simulink model "AOM_new"  (R2023a)
settings: Solver=ode4  StartTime=0.0  StopTime=5  FixedStep=0.001  RelTol=1e-3
values from neighbouring files (symbols this model uses):
  dot_X0 = initial_condition(4:5)    [actor_critic.m]
  trajectory = zeros(4, length(all_new))    [actor_critic.m]
  X0 = initial_condition(1:2)    [actor_critic.m]
libraries: rllib x1
settings Model: Creator=Ali  LastModifiedBy=Ali

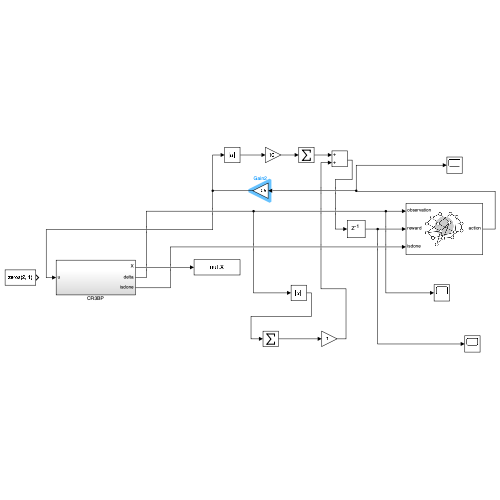
[thumbnail: Simulink's stored preview of the top-level diagram]
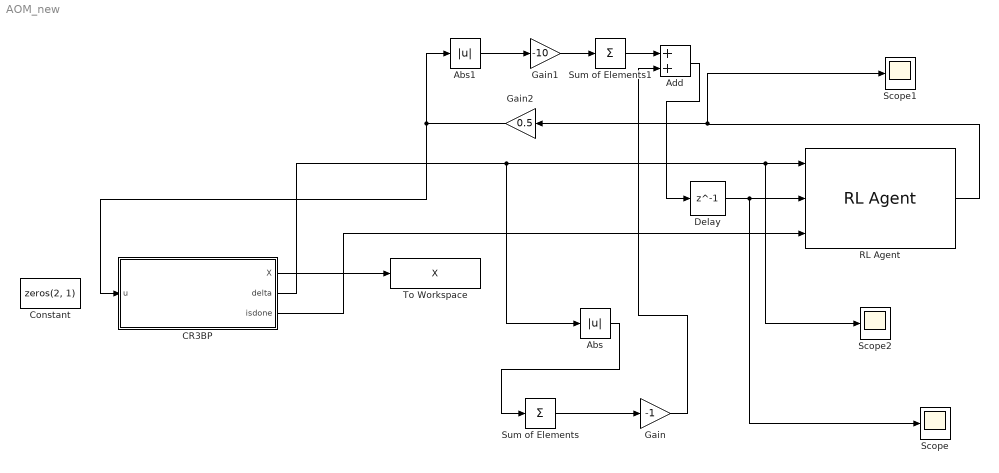
== system AOM_new ==
  Abs : Abs  SaturateOnIntegerOverflow=off
  Abs1 : Abs  SaturateOnIntegerOverflow=off
  Add : Sum
  CR3BP : Subsystem
  Constant : Constant  Value=zeros(2, 1)
  Delay : Delay  DelayLength=1
  Gain : Gain  Gain=-1
  Gain1 : Gain  Gain=-10
  Gain2 : Gain  Gain=0.5
  RL Agent : rllib/RL Agent  Agent=agent2_Trained_3  ExternalActionAsInput=off  ProvideLastAction=off  ProvideCumRwd=off  TreatAsDirectFeedthrough=on  UseStrictObservationDataTypes=off
  Scope : Scope
  Scope1 : Scope
  Scope2 : Scope
  Sum of Elements : Sum  Inputs=+
  Sum of Elements1 : Sum  Inputs=+
  To Workspace : ToWorkspace  VariableName=X  SaveFormat=Timeseries  SampleTime=-1
  wires:
  CR3BP/1(X) -> To Workspace/1
  CR3BP/3(isdone) -> RL Agent/3
  RL Agent/1 -> Gain2/1, Scope1/1
  CR3BP/2(delta) -> Abs/1, Scope2/1, RL Agent/1
  Abs/1 -> Sum of Elements/1
  Sum of Elements/1 -> Gain/1
  Gain/1 -> Add/2
  Delay/1 -> Scope/1, RL Agent/2
  Abs1/1 -> Gain1/1
  Add/1 -> Delay/1
  Sum of Elements1/1 -> Add/1
  Gain1/1 -> Sum of Elements1/1
  Gain2/1 -> CR3BP/1(u), Abs1/1

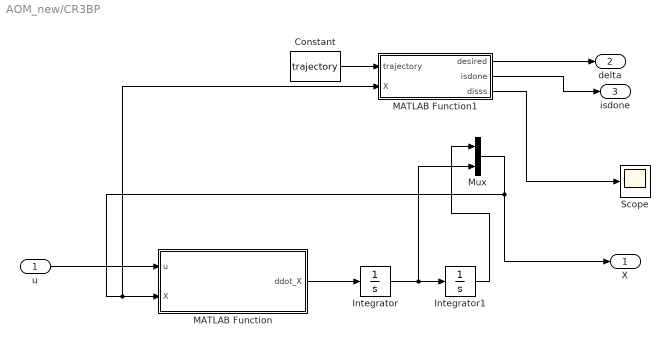
== system AOM_new/CR3BP ==
  u : Inport
  Constant : Constant  Value=trajectory
  Integrator : Integrator  InitialCondition=dot_X0
  Integrator1 : Integrator  InitialCondition=X0
  MATLAB Function : MATLAB Function  TreatAsAtomicUnit=on
  MATLAB Function1 : MATLAB Function  TreatAsAtomicUnit=on
  Mux : Mux  Inputs=2
  Scope : Scope
  X : Outport
  delta : Outport  Port=2
  isdone : Outport  Port=3
  wires:
  u/1 -> MATLAB Function/1(u)
  Integrator1/1 -> Mux/1
  Integrator/1 -> Mux/2, Integrator1/1
  MATLAB Function/1(ddot_X) -> Integrator/1
  Mux/1 -> X/1, MATLAB Function1/2(X), MATLAB Function/2(X)
  Constant/1 -> MATLAB Function1/1(trajectory)
  MATLAB Function1/1(desired) -> delta/1
  MATLAB Function1/2(isdone) -> isdone/1
  MATLAB Function1/3(disss) -> Scope/1

== matlab function AOM_new/CR3BP/MATLAB Function1 ==
  data: trajectory input; desired output size=[4, 1]; X input; isdone output; disss output
function [desired, isdone, disss] = fcn(trajectory, X)



xy = X(1:2);
distance = ((trajectory(1:2, :) - xy).^2);
dist = sum(distance);
dist = dist';
index = dist==min(dist);
answer = trajectory(:, index);

desired = reshape(answer, [4, 1]) - reshape(X, [4, 1]);
desired = desired * 100;

isdone = false;
final_point = trajectory(1:2, end);
disss = sqrt(sum((xy - final_point).^2));
if disss <= 0.005
    isdone = true;
end

== matlab function AOM_new/CR3BP/MATLAB Function ==
  data: u input; ddot_X output; X input
function ddot_X = fcn(u, X)

mu = 0.012277471;

a_x = u(1);
a_y = u(2);

% Positions
x = X(1);
y = X(2);
z = 0;
% Velocities
xdot = X(3);
ydot = X(4);

% distances from particle to primaries
r1 = sqrt((x+mu)^2 + y^2 + z^2); 
r2 = sqrt((x-1+mu)^2 + y^2 + z^2); 

% Accelerations 
xddot = 2*ydot + x -(1-mu)*((x+mu)/(r1^3)) - mu*(x-1+mu)/(r2^3) + a_x;
yddot = -2*xdot + y - (1-mu)*(y/(r1^3)) - mu*(y)/(r2^3) + a_y;

ddot_X = [xddot; yddot];
